simulink model "sim_punto_6"  (R2021b)
settings: Solver=ode45  StartTime=0.0  StopTime=tsim  RelTol=1e-3  EnableMultiTasking=on
values from neighbouring files (symbols this model uses):
  A = [0 1 0 0 0 0 0 0 0 0 0 0 ... (first row only)    [punto6.m]
  B = [0; 0; 0; 0; 0; 0; 0; 0; 0; 0; 0; 1]    [punto6.m]
  B_noise = [B ones(size(B,1),1)]    [punto6.m]
  C = [1 0 0 0 0 0 0 0 0 0 0 0]    [punto6.m]
  C_states = eye(12)    [punto6.m]
  D = 0    [punto6.m]
  D_noise = [D_states zeros(size(D_states,1),1)]    [punto6.m]
  N3 = 27    [punto6.m]
  NK = 0    [punto6.m]
  Q = [1+q 0 0 0 0 0 0 0 0 0 0 0 ... (first row only)    [punto6.m]
  R = r    (= 1e-05)    [punto6.m]
  RK = 10*QK(1)    [punto6.m]
  S = [0 0 0 0 0 0 0 0 0 0 0 0 ... (first row only)    [punto6.m]
  Ts = 0.1    [punto6.m]
  U_max = 15    [punto6.m]
  U_min = -15    [punto6.m]
  Ubar = inv(g)*Ybar    [punto6.m]
  umax = 15    [punto6.m]
  umin = -15    [punto6.m]
  x0 = [0 0 0 0 0 0 0 0 0 0 0 0]'    [punto6.m]
  x0K = 1.5*x0    [punto6.m]
  Xbar = -inv(A) * B * Ubar    [punto6.m]
  Xbar_disc = (eye(12)- A)^-1*B*Ubar    [punto6.m]
  xmax = [repmat(xmax,N,1)]    [mympc.m]    (also in punto6.m = [10 0 10 0 10 0 10 0 10 0 10 0]')
  xmin = [repmat(xmin,N,1)]    [mympc.m]    (also in punto6.m = [-10 0 -10 0 -10 0 -10 0 -10 0 -10 0]')
undefined symbols (not defined in the file or in its folder): Discrete, K_disc, mympc, Time
libraries: simulink x4, ctrlSharedLib x2
settings Model: Creator=Administrator  LastModifiedBy=danie
settings SolverCC: AlgebraicLoopSolver=TrustRegion
settings DataIOCC: LimitDataPoints=on  SaveFormat=Array  SignalLoggingSaveFormat=ModelDataLogs  ReturnWorkspaceOutputs=off
settings OptimizationCC: ExpressionDepthLimit=2147483647  InitFltsAndDblsToZero=on  LifeSpan=inf
settings DebuggingCC: UnderspecifiedInitializationDetection=Classic  MergeDetectMultiDrivingBlocksExec=none  SolverPrmCheckMsg=warning  FcnCallInpInsideContextMsg=warning  StateNameClashWarn=warning  SFUnexpectedBacktrackingDiag=warning  SFNoUnconditionalDefaultTransitionDiag=warning  SFExecutionAtInitializationDiag=none  ArithmeticOperatorsInVariantConditions=warning
settings HardwareCC: ProdBitPerPointer=32  ProdBitPerSizeT=32  ProdBitPerPtrDiffT=32  ProdLargestAtomicFloat=None  ProdIntDivRoundTo=Undefined  ProdEndianess=Unspecified  ProdWordSize=32  ProdHWDeviceType=32-bit Generic
settings ModelReferenceCC: PropagateSignalLabelsOutOfModel=off
settings SFSimCC: SimUseLocalCustomCode=off  CustomCodeUndefinedFunction=UseInterfaceOnly
settings RTWCC: RTWUseLocalCustomCode=off  DLArmComputeVersion=20.02.1
settings CodeAppCC: StateflowObjectComments=on
settings GRTTargetCC: TargetLangStandard=C89/C90 (ANSI)  CombineOutputUpdateFcns=off  GRTInterface=on
settings ConfigComp: CovMetricSettings=dw  CovSaveCumulativeToWorkspaceVar=on  CovSaveSingleToWorkspaceVar=on  CovExternalEMLEnable=off  CovSFcnEnable=off

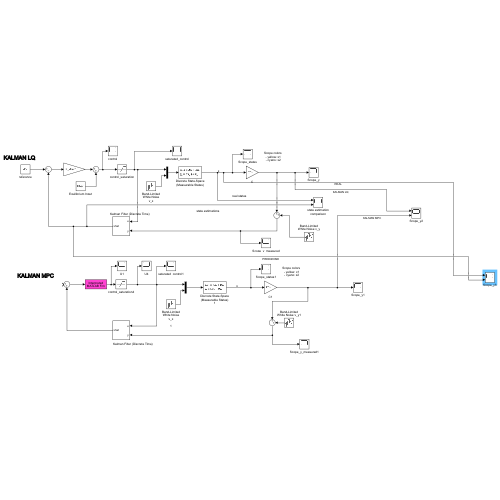
[thumbnail: Simulink's stored preview of the top-level diagram]
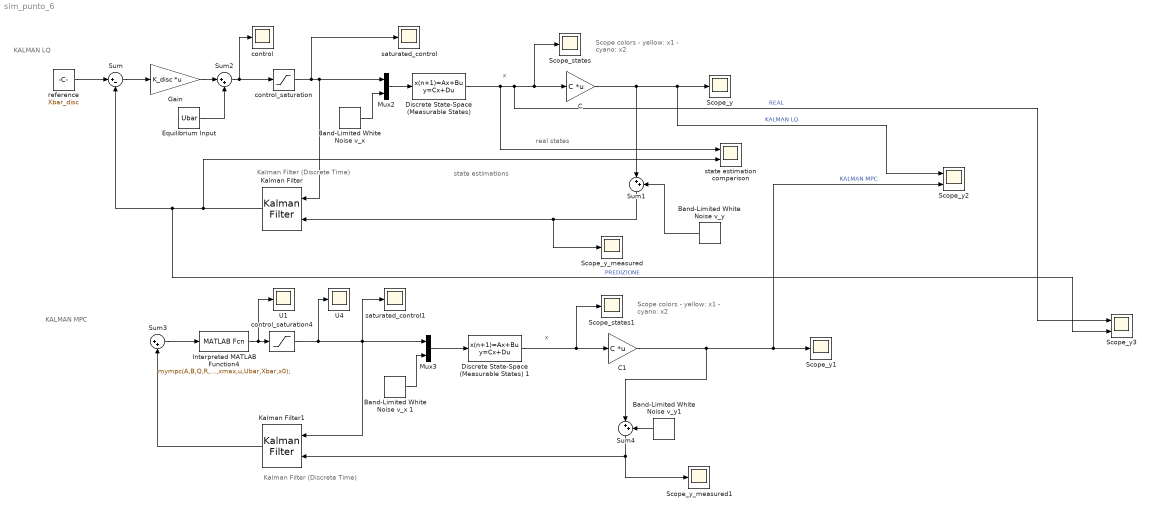
== system sim_punto_6 ==
  note: KALMAN LQ
  note: Kalman Filter (Discrete Time)
  note: real states
  note: state estimations
  note: x
  note: Scope colors
      | - yellow: x1
      | - cyano: x2
  note: KALMAN MPC
  note: x
  note: Kalman Filter (Discrete Time)
  note: Scope colors
      | - yellow: x1
      | - cyano: x2
  "Band-Limited White Noise v_x " : simulink/Sources/Band-Limited White Noise  Cov=power_vx  Ts=Ts  seed=[23341]
  Band-Limited White Noise v_x 1 : simulink/Sources/Band-Limited White Noise  Cov=power_vx  Ts=Ts  seed=[23341]
  Band-Limited White Noise v_y : simulink/Sources/Band-Limited White Noise  Cov=power_vy  Ts=Ts  seed=[1258]
  Band-Limited White Noise v_y1 : simulink/Sources/Band-Limited White Noise  Cov=power_vy  Ts=Ts  seed=[1258]
  C : Gain  Gain=C  Multiplication=Matrix(K*u)
  C1 : Gain  Gain=C  Multiplication=Matrix(K*u)
  "Discrete State-Space (Measurable States) " : DiscreteStateSpace  A=A  B=B_noise  C=C_states  D=D_noise  InitialCondition=x0  SampleTime=Ts
  Discrete State-Space (Measurable States) 1 : DiscreteStateSpace  A=A  B=B_noise  C=C_states  D=D_noise  InitialCondition=x0  SampleTime=Ts
  Equilibrium Input : Constant  Value=Ubar
  Gain : Gain  Gain=K_disc  Multiplication=Matrix(K*u)
  Interpreted MATLAB Function4 : MATLABFcn  MATLABFcn=mympc(A,B,Q,R,S,N3,umin,umax,xmin,xmax,u,Ubar,Xbar,x0);  OutputDimensions=1
  Kalman Filter : ctrlSharedLib/Kalman Filter  TimeDomain=Discrete-Time  UseCurrentEstimator=on  ModelSource=Individual A, B, C, D matrices  ModelSourceVariable=ss(0.95,1,1,0,1)  A=A  B=B  C=C  D=D  NumberOfStates=1  NumberOfInputs=1  NumberOfOutputs=1  InitialEstimateSource=Dialog  X0=x0K  P0=10  UseK=off  UseGH=off  NumberOfProcessNoiseInputs=1  G=1  TimeInvariantG=on  H=0  TimeInvariantH=on  Q=QK  TimeInvariantQ=on  R=RK  TimeInvariantR=on  N=NK  TimeInvariantN=on  AddInputPort=on  AddEnablePort=off  OutputEstimatedY=off  OutputP=off  Ts=Ts
  Kalman Filter1 : ctrlSharedLib/Kalman Filter  TimeDomain=Discrete-Time  UseCurrentEstimator=on  ModelSource=Individual A, B, C, D matrices  ModelSourceVariable=ss(0.95,1,1,0,1)  A=A  B=B  C=C  D=D  NumberOfStates=1  NumberOfInputs=1  NumberOfOutputs=1  InitialEstimateSource=Dialog  X0=x0K  P0=10  UseK=off  UseGH=off  NumberOfProcessNoiseInputs=1  G=1  TimeInvariantG=on  H=0  TimeInvariantH=on  Q=QK  TimeInvariantQ=on  R=RK  TimeInvariantR=on  N=NK  TimeInvariantN=on  AddInputPort=on  AddEnablePort=off  OutputEstimatedY=off  OutputP=off  Ts=Ts
  Mux2 : Mux  Inputs=2
  Mux3 : Mux  Inputs=2
  Scope_states : Scope
  Scope_states1 : Scope
  Scope_y : Scope
  Scope_y1 : Scope
  Scope_y2 : Scope  NumInputPorts=2
  Scope_y3 : Scope  NumInputPorts=2
  Scope_y_measured : Scope
  Scope_y_measured1 : Scope
  Sum : Sum  Inputs=|+-
  Sum{1..4} (4 alike) : Sum  Inputs=|++
  U1 : Scope
  U4 : Scope
  control : Scope
  control_saturation : Saturate  UpperLimit=U_max  LowerLimit=U_min
  control_saturation4 : Saturate  UpperLimit=umax  LowerLimit=umin
  reference : Constant  Value=Xbar_disc
  saturated_control : Scope
  saturated_control1 : Scope
  "state estimation comparison " : Scope  NumInputPorts=2
  wires:
  reference/1 -> Sum/1
  Sum/1 -> Gain/1
  "Discrete State-Space (Measurable States) "/1 -> "state estimation comparison "/1, Scope_y3/1, Scope_states/1, C/1  "REAL"
  C/1 -> Sum1/1, Scope_y2/1, Scope_y/1  "KALMAN LQ"
  control_saturation/1 -> Kalman Filter/1, Mux2/1, saturated_control/1
  Mux2/1 -> "Discrete State-Space (Measurable States) "/1
  Sum1/1 -> Scope_y_measured/1, Kalman Filter/2
  Gain/1 -> Sum2/1
  Sum2/1 -> control/1, control_saturation/1
  Equilibrium Input/1 -> Sum2/2
  Kalman Filter/1 -> Scope_y3/2, Sum/2, "state estimation comparison "/2  "PREDIZIONE"
  Band-Limited White Noise v_y/1 -> Sum1/2
  "Band-Limited White Noise v_x "/1 -> Mux2/2
  control_saturation4/1 -> U4/1, Kalman Filter1/1, saturated_control1/1, Mux3/1
  Discrete State-Space (Measurable States) 1/1 -> Scope_states1/1, C1/1
  Sum4/1 -> Scope_y_measured1/1, Kalman Filter1/2
  Mux3/1 -> Discrete State-Space (Measurable States) 1/1
  Sum3/1 -> Interpreted MATLAB Function4/1
  Band-Limited White Noise v_y1/1 -> Sum4/2
  Band-Limited White Noise v_x 1/1 -> Mux3/2
  Kalman Filter1/1 -> Sum3/2
  C1/1 -> Scope_y2/2, Scope_y1/1, Sum4/1  "KALMAN MPC"
  Interpreted MATLAB Function4/1 -> U1/1, control_saturation4/1
